simulink library "lib_accessory2"  (Simulink 10.1)
settings: Solver=VariableStepAuto  StartTime=0.0  StopTime=10.0  RelTol=1e-3
undefined symbols (not defined in the file or in its folder): acc_dcdc_eff, acc_elec_eff, acc_elec_efficiency, acc_elec_pwr, acc_mech_eff, acc_mech_pwr, acc_mech_trq, amb_tmp, ess_on, fc_on, map_spd, max_pwr, tc_gc_to_fc_ratio, time_step, vc_idle_bool, vc_idle_spd, vinf
undefined symbols (not defined in the file): acc_abc_dutycycle, acc_abc_init, acc_ac_dutycycle, acc_ac_init, acc_acdc_inverter_eff, acc_alt_init, acc_ef_dutycycle, acc_ef_init, acc_op_dutycycle, acc_op_init, acc_ps_dutycycle, acc_ps_init, acc_sindafile, acc_wp_dutycycle, acc_wp_init, generalName, logFlag
libraries: lib_cosimulation x29, $bdroot x15, lib_outputs x11, simulink3 x10, lib_accessory x8, lib_etc x2
(part 1 of 5)
settings Model: Creator=sateeshk  LastModifiedBy=sateeshk  ModifiedComment=abrooker -- Fri Jun 21 11:06:39 2002 -- Version 1.443
settings Model: ModifiedHistory=|
  | abrooker -- Fri Jun 21 11:06:39 2002 -- Version 1.443
  | 
  | 
  | abrooker -- Fri Jun 21 11:06:32 2002 -- Version 1.442
  | 
  | 
  | abrooker -- Fri Jun 21 11:03:06 2002 -- Version 1.441
  | 
  | 
  | abrooker -- Fri Jun 21 08:18:53 2002 -- Version 1.440
  | 
  | 
  | abrooker -- Fri Jun 21 08:07:14 2002 -- Version 1.439
  | 
  | 
  | abrooker -- Fri Jun 21 07:53:07 2002 -- Version 1.438
  | 
  | 
  | abrooker -- Thu Jun 20 15:33:10 2002 -- Version 1.437
  | 
  | 
  | abrooker -- Thu Jun 20 15:32:18 2002 -- Version 1.436
  | 
  | 
  | mokeefe -- Wed May 22 16:23:29 2002 -- Version 1.435
  | changed SindaTransAC model to take 5 outputs
  | 
  | mokeefe -- Thu Apr 18 08:24:09 2002 -- Version 1.434
  | saving the model:
  | o "without the model browser open"
  | o with only top-level screen visible
  | o with "fit to view" enabled
  | o with "status bar" off and "toolbar" off
  | o with "prompt to update model history with each save" on
  | 
  | tmarkel -- Mon Apr 15 11:38:46 2002 -- Version 1.428
  | 
  | 
  | tmarkel -- Mon Apr 15 11:38:46 2002 -- Version 1.428
  | 
  | 
  | tmarkel -- Mon Apr 15 11:38:36 2002 -- Version 1.427
  | 
  | 
  | mokeefe -- Mon Apr 15 11:36:55 2002 -- Version 1.426
  | added acc_sindafile variable into the SindaTransAC model
  | 
  | 
  | 
  | 
  | 
  | mokeefe -- Mon Apr 15 11:30:03 2002 -- Version 1.424
  | adding a feature to the sinda fluint s-function so that user can pass in the path to their executable file (*.im) function
  | 
  | 
  | abrooker -- Thu Apr 11 17:26:32 2002 -- Version 1.423
  | added vc_idle_bool in minimum fc shaft speed for stop/start:  otherwise
  | 
  | mokeefe -- Wed Apr 03 17:17:08 2002 -- Version 1.422
  | checked the configurable sub-system option for SindaTransAC
  | 
  | abrooker -- Tue Apr 02 08:21:35 2002 -- Version 1.421
  | 
  | 
  | abrooker -- Tue Apr 02 08:16:39 2002 -- Version 1.420
  | 
  | 
  | mokeefe -- Fri Mar 29 16:21:02 2002 -- Version 1.419
  | 
  | 
  | mokeefe -- Fri Mar 29 16:18:34 2002 -- Version 1.418
  | added SindaTransAC Sinda/Fluint cosim aux. model (transient air condition modeling)
  | 
  | mokeefe -- Fri Mar 29 09:01:44 2002 -- Version 1.417
  | 
  | 
  | mokeefe -- Fri Mar 29 09:00:29 2002 -- Version 1.416
  | 
  | 
  | mokeefe -- Fri Mar 29 08:55:21 2002 -- Version 1.415
  | 
  | 
  | mokeefe -- Fri Mar 29 08:54:32 2002 -- Version 1.414
  | 
  | 
  | mokeefe -- Fri Mar 29 08:34:07 2002 -- Version 1.413
  | 
  | 
  | mokeefe -- Fri Mar 29 08:33:22 2002 -- Version 1.412
  | rearranging the library for aesthetic purposes =)
  | 
  | mokeefe -- Fri Mar 29 08:27:44 2002 -- Version 1.411
  | took out two of the mechanical accessory options that will probably not be used (the same functionality is available with the remaining blocks). These blocks moved to the development subsystem for storage.
  | 
  | abrooker -- Thu Mar 28 16:18:46 2002 -- Version 1.410
  | (mokeefe) changed the Mechanical Accessory Load Driveline Block to use memory blocks for torque and power estimation (as opposed to two calculations)
  | 
  | abrooker -- Thu Mar 28 12:33:24 2002 -- Version 1.409
  | 
  | 
  | abrooker -- Thu Mar 28 12:25:41 2002 -- Version 1.408
  | 
  | 
  | abrooker -- Thu Mar 28 12:08:36 2002 -- Version 1.407
  | 
  | 
  | abrooker -- Thu Mar 28 12:04:18 2002 -- Version 1.406
  | 
  | 
  | abrooker -- Thu Mar 28 08:53:24 2002 -- Version 1.405
  | 
  | 
  | abrooker -- Thu Mar 28 08:49:44 2002 -- Version 1.404
  | 
  | 
  | mokeefe -- Wed Mar 27 07:38:24 2002 -- Version 1.403
  | 
  | 
  | mokeefe -- Wed Mar 27 07:37:49 2002 -- Version 1.402
  | added a masked variable (acc_max_spd) to the mechanical accessory loads library
  | 
  | mokeefe -- Wed Mar 20 10:22:56 2002 -- Version 1.401
  | changed the pictures for the configurable subsystem blocks to differentiate from the driveline blocks
  | 
  | mokeefe -- Tue Mar 12 13:44:43 2002 -- Version 1.400
  | 
  | 
  | mokeefe -- Tue Mar 12 13:36:01 2002 -- Version 1.399
  | cleaned up the library and reorganized block positions
  | 
  | 
  | mokeefe -- Tue Mar 12 13:34:33 2002 -- Version 1.398
  | 
  | 
  | mokeefe -- Tue Mar 12 13:34:15 2002 -- Version 1.397
  | 
  | 
  | mokeefe -- Tue Mar 12 13:29:31 2002 -- Version 1.396
  | 
  | 
  | mokeefe -- Tue Mar 12 13:25:46 2002 -- Version 1.395
  | 
  | 
  | mokeefe -- Tue Mar 12 13:09:55 2002 -- Version 1.394
  | changed the variable mechanical loads to include a water pump
  | 
  | mokeefe -- Tue Mar 12 12:07:07 2002 -- Version 1.393
  | 
  | 
  | mokeefe -- Tue Mar 12 12:06:03 2002 -- Version 1.392
  | 
  | 
  | mokeefe -- Tue Mar 12 12:04:31 2002 -- Version 1.391
  | 
  | 
  | mokeefe -- Tue Mar 12 11:59:22 2002 -- Version 1.390
  | 
  | 
  | mokeefe -- Tue Mar 12 11:54:25 2002 -- Version 1.389
  | changing the way that data signals are recorded (especially for the variable mechanical loads blocks--see SubLibraries/variable mechanical load --simulink implementation--)
  | 
  | mokeefe -- Fri Mar 08 07:13:02 2002 -- Version 1.388
  | added the tag acc_mech_pwr_est as a global tag to Mechanical Accessory Loads v2 <acc>
  | 
  | mokeefe -- Mon Mar 04 07:28:37 2002 -- Version 1.387
  | 
  | 
  | mokeefe -- Mon Mar 04 07:27:09 2002 -- Version 1.386
  | 
  | 
  | mokeefe -- Mon Mar 04 07:24:49 2002 -- Version 1.385
  | changed the mechanical accessory torque back to a simple version
  | 
  | mokeefe -- Fri Mar 01 16:40:21 2002 -- Version 1.384
  | 
  | 
  | mokeefe -- Fri Mar 01 16:37:19 2002 -- Version 1.383
  | 
  | 
  | mokeefe -- Fri Mar 01 15:08:33 2002 -- Version 1.382
  | 
  | 
  | mokeefe -- Fri Mar 01 12:12:06 2002 -- Version 1.381
  | 
  | 
  | mokeefe -- Fri Mar 01 12:10:27 2002 -- Version 1.380
  | 
  | 
  | mokeefe -- Fri Mar 01 11:39:14 2002 -- Version 1.379
  | 
  | 
  | mokeefe -- Fri Mar 01 11:20:41 2002 -- Version 1.378
  | 
  | 
  | mokeefe -- Fri Mar 01 10:50:57 2002 -- Version 1.377
  | 
  | 
  | mokeefe -- Fri Mar 01 10:18:24 2002 -- Version 1.376
  | 
  | 
  | mokeefe -- Fri Mar 01 10:16:01 2002 -- Version 1.375
  | 
  | 
  | mokeefe -- Fri Mar 01 10:13:39 2002 -- Version 1.374
  | 
  | 
  | mokeefe -- Fri Mar 01 09:58:45 2002 -- Version 1.373
  | 
  | 
  | mokeefe -- Fri Mar 01 09:31:13 2002 -- Version 1.372
  | 
  | 
  | mokeefe -- Fri Mar 01 09:30:34 2002 -- Version 1.371
  | 
  | 
  | mokeefe -- Fri Mar 01 09:00:19 2002 -- Version 1.370
  | 
  | 
  | mokeefe -- Fri Mar 01 08:27:00 2002 -- Version 1.369
  | 
  | 
  | mokeefe -- Fri Mar 01 08:04:14 2002 -- Version 1.368
  | 
  | 
  | mokeefe -- Thu Feb 28 08:51:52 2002 -- Version 1.367
  | 
  | 
  | mokeefe -- Thu Feb 28 08:48:14 2002 -- Version 1.366
  | 
  | 
  | mokeefe -- Thu Feb 28 08:21:55 2002 -- Version 1.365
  | 
  | 
  | mokeefe -- Thu Feb 28 08:20:46 2002 -- Version 1.364
  | adding an on/off flag for auxiliary systems to account for "engine off" states
  | 
  | mokeefe -- Thu Feb 28 08:10:24 2002 -- Version 1.363
  | 
  | 
  | mokeefe -- Wed Feb 27 14:38:39 2002 -- Version 1.362
  | 
  | 
  | mokeefe -- Wed Feb 27 14:34:06 2002 -- Version 1.361
  | 
  | 
  | mokeefe -- Wed Feb 27 14:33:33 2002 -- Version 1.360
  | 
  | 
  | mokeefe -- Wed Feb 27 14:29:19 2002 -- Version 1.359
  | 
  | 
  | mokeefe -- Wed Feb 27 14:12:33 2002 -- Version 1.358
  | 
  | 
  | mokeefe -- Wed Feb 27 14:11:56 2002 -- Version 1.357
  | 
  | 
  | mokeefe -- Wed Feb 27 14:06:17 2002 -- Version 1.356
  | 
  | 
  | mokeefe -- Wed Feb 27 14:04:01 2002 -- Version 1.355
  | added a "version 2" to mechanical auxiliary loads library which has a workaround that takes in the fc_spd_est instead of fc_spd_out_a--this enables vehicles to have an exact match between ADVISOR v3.2 and v2002
  | 
  | mokeefe -- Wed Feb 27 09:55:44 2002 -- Version 1.354
  | 
  | 
  | mokeefe -- Wed Feb 27 09:53:42 2002 -- Version 1.
  | 
  | mokeefe -- Tue Feb 26 15:16:41 2002 -- Version 1.352
  | 
  | 
  | mokeefe -- Tue Feb 26 14:01:11 2002 -- Version 1.351
  | 
  | 
  | mokeefe -- Tue Feb 26 13:25:47 2002 -- Version 1.350
  | 
  | 
  | mokeefe -- Tue Feb 26 10:40:53 2002 -- Version 1.349
  | 
  | 
  | mokeefe -- Mon Feb 25 16:05:53 2002 -- Version 1.348
  | 
  | 
  | mokeefe -- Mon Feb 25 15:35:04 2002 -- Version 1.347
  | 
  | 
  | mokeefe -- Mon Feb 25 15:33:00 2002 -- Version 1.346
  | 
  | 
  | mokeefe -- Mon Feb 25 15:26:23 2002 -- Version 1.345
  | 
  | 
  | mokeefe -- Mon Feb 25 15:24:36 2002 -- Version 1.344
  | 
  | 
  | mokeefe -- Mon Feb 25 15:23:19 2002 -- Version 1.343
  | 
  | 
  | mokeefe -- Mon Feb 25 15:19:58 2002 -- Version 1.342
  | 
  | 
  | mokeefe -- Mon Feb 25 15:17:22 2002 -- Version 1.341
  | 
  | 
  | mokeefe -- Mon Feb 25 15:04:08 2002 -- Version 1.340
  | 
  | 
  | mokeefe -- Mon Feb 25 14:59:43 2002 -- Version 1.339
  | 
  | 
  | mokeefe -- Mon Feb 25 14:50:11 2002 -- Version 1.338
  | 
  | 
  | mokeefe -- Mon Feb 25 14:37:23 2002 -- Version 1.337
  | 
  | 
  | mokeefe -- Mon Feb 25 14:24:02 2002 -- Version 1.336
  | 
  | 
  | mokeefe -- Mon Feb 25 14:19:40 2002 -- Version 1.335
  | 
  | 
  | mokeefe -- Mon Feb 25 14:14:18 2002 -- Version 1.334
  | 
  | 
  | mokeefe -- Mon Feb 25 14:09:13 2002 -- Version 1.333
  | 
  | 
  | mokeefe -- Mon Feb 25 13:38:54 2002 -- Version 1.332
  | 
  | 
  | mokeefe -- Mon Feb 25 13:38:02 2002 -- Version 1.331
  | 
  | 
  | mokeefe -- Wed Feb 20 09:52:02 2002 -- Version 1.330
  | 
  | 
  | mokeefe -- Wed Feb 20 09:49:29 2002 -- Version 1.329
  | changed the acc_mech_trq_a, acc_mech_pwr_a, acc_mech_trq_r, acc_mech_pwr_r, acc_elec_pwr_a, acc_elec_pwr_r GOTO blocks to global scope.
  | 
  | mokeefe -- Wed Feb 20 09:47:28 2002 -- Version 1.328
  | 
  | 
  | mokeefe -- Wed Feb 20 09:46:46 2002 -- Version 1.327
  | 
  | 
  | mokeefe -- Wed Feb 20 07:42:37 2002 -- Version 1.326
  | 
  | 
  | mokeefe -- Wed Feb 20 07:42:12 2002 -- Version 1.325
  | 
  | 
  | mokeefe -- Wed Feb 20 07:41:46 2002 -- Version 1.324
  | 
  | 
  | mokeefe -- Tue Feb 19 16:34:31 2002 -- Version 1.323
  | 
  | 
  | mokeefe -- Tue Feb 19 16:31:37 2002 -- Version 1.322
  | 
  | 
  | mokeefe -- Tue Feb 19 16:28:38 2002 -- Version 1.321
  | changed the accessory GOTO tags to global scope in Electrical Accessory Loads
  | 
  | mokeefe -- Tue Feb 19 16:14:33 2002 -- Version 1.320
  | first release to RCS
  | 
  | mokeefe -- Tue Feb 19 16:12:28 2002 -- Version 1.319
  | 
  | 
  | mokeefe -- Tue Feb 19 16:06:11 2002 -- Version 1.318
  | 
  | 
  | mokeefe -- Tue Feb 19 16:02:32 2002 -- Version 1.317
  | 
  | 
  | mokeefe -- Tue Feb 19 15:58:43 2002 -- Version 1.316
  | 
  | 
  | mokeefe -- Tue Feb 19 15:55:41 2002 -- Version 1.315
  | 
  | 
  | mokeefe -- Tue Feb 19 15:53:46 2002 -- Version 1.314
  | 
  | 
  | mokeefe -- Tue Feb 19 15:49:12 2002 -- Version 1.313
  | 
  | 
  | mokeefe -- Tue Feb 19 15:42:48 2002 -- Version 1.312
  | 
  | 
  | mokeefe -- Tue Feb 19 15:41:05 2002 -- Version 1.311
  | 
  | 
  | mokeefe -- Tue Feb 19 15:38:40 2002 -- Version 1.310
  | 
  | 
  | mokeefe -- Tue Feb 19 15:28:06 2002 -- Version 1.309
  | 
  | 
  | mokeefe -- Tue Feb 19 15:18:02 2002 -- Version 1.308
  | 
  | 
  | mokeefe -- Tue Feb 19 14:53:21 2002 -- Version 1.307
  | 
  | 
  | mokeefe -- Tue Feb 19 14:46:24 2002 -- Version 1.306
  | 
  | 
  | mokeefe -- Tue Feb 19 14:20:08 2002 -- Version 1.305
  | 
  | 
  | mokeefe -- Tue Feb 19 14:15:36 2002 -- Version 1.304
  | 
  | 
  | mokeefe -- Tue Feb 19 13:24:42 2002 -- Version 1.303
  | 
  | 
  | mokeefe -- Tue Feb 19 13:17:05 2002 -- Version 1.302
  | 
  | 
  | mokeefe -- Tue Feb 19 13:11:20 2002 -- Version 1.301
  | 
  | 
  | mokeefe -- Tue Feb 19 11:29:38 2002 -- Version 1.300
  | 
  | 
  | mokeefe -- Tue Feb 19 11:24:45 2002 -- Version 1.299
  | adding electrical accessory block
  | 
  | 
  | mokeefe -- Tue Feb 19 10:53:36 2002 -- Version 1.298
  | 
  | 
  | mokeefe -- Tue Feb 19 10:19:54 2002 -- Version 1.297
  | added electrical accessory loads block
  | 
  | 
  | mokeefe -- Thu Feb 14 17:56:03 2002 -- Version 1.296
  | 
  | 
  | mokeefe -- Thu Feb 14 17:54:33 2002 -- Version 1.295
  | 
  | 
  | mokeefe -- Thu Feb 14 17:51:07 2002 -- Version 1.294
  | 
  | 
  | mokeefe -- Thu Feb 14 17:49:19 2002 -- Version 1.293
  | changing the way that data is "logged" to displays and scopes vs. workspace on some components that I expect will have to be used multiple times... (a workaround for now)
  | 
  | mokeefe -- Thu Feb 14 17:21:35 2002 -- Version 1.292
  | 
  | 
  | mokeefe -- Thu Feb 14 16:55:33 2002 -- Version 1.291
  | 
  | 
  | mokeefe -- Thu Feb 14 16:21:30 2002 -- Version 1.290
  | 
  | 
  | mokeefe -- Thu Feb 14 16:19:08 2002 -- Version 1.289
  | 
  | 
  | mokeefe -- Thu Feb 14 16:17:00 2002 -- Version 1.288
  | 
  | 
  | mokeefe -- Thu Feb 14 16:15:50 2002 -- Version 1.287
  | 
  | 
  | mokeefe -- Thu Feb 14 16:14:24 2002 -- Version 1.286
  | 
  | 
  | mokeefe -- Thu Feb 14 16:13:43 2002 -- Version 1.285
  | 
  | 
  | mokeefe -- Thu Feb 14 15:43:46 2002 -- Version 1.284
  | 
  | 
  | mokeefe -- Thu Feb 14 15:42:22 2002 -- Version 1.283
  | 
  | 
  | mokeefe -- Thu Feb 14 15:31:24 2002 -- Version 1.282
  | 
  | 
  | mokeefe -- Thu Feb 14 15:26:13 2002 -- Version 1.281
  | 
  | 
  | mokeefe -- Thu Feb 14 15:25:37 2002 -- Version 1.280
  | 
  | 
  | mokeefe -- Thu Feb 14 15:19:19 2002 -- Version 1.279
  | 
  | 
  | mokeefe -- Thu Feb 14 15:10:41 2002 -- Version 1.278
  | 
  | 
  | mokeefe -- Thu Feb 14 14:28:51 2002 -- Version 1.277
  | 
  | 
  | mokeefe -- Thu Feb 14 14:26:34 2002 -- Version 1.276
  | 
  | 
  | mokeefe -- Thu Feb 14 10:50:49 2002 -- Version 1.275
  | 
  | 
  | mokeefe -- Thu Feb 14 10:47:05 2002 -- Version 1.274
  | 
  | 
  | mokeefe -- Thu Feb 14 10:40:54 2002 -- Version 1.273
  | 
  | 
  | mokeefe -- Thu Feb 14 10:23:01 2002 -- Version 1.272
  | 
  | 
  | mokeefe -- Thu Feb 14 10:05:05 2002 -- Version 1.271
  | 
  | 
  | mokeefe -- Thu Feb 14 09:56:25 2002 -- Version 1.270
  | 
  | 
  | mokeefe -- Thu Feb 14 09:55:54 2002 -- Version 1.269
  | changed the "signal width" parameters of blocks such that they work correctly
  | 
  | mokeefe -- Thu Feb 14 09:54:47 2002 -- Version 1.268
  | 
  | 
  | mokeefe -- Thu Feb 14 09:51:13 2002 -- Version 1.267
  | 
  | 
  | mokeefe -- Thu Feb 14 08:58:02 2002 -- Version 1.266
  | 
  | 
  | mokeefe -- Thu Feb 14 08:39:00 2002 -- Version 1.265
  | changed the port width in alternator block back to dynamically sized
  | 
  | 
  | mokeefe -- Thu Feb 14 08:06:18 2002 -- Version 1.264
  | 
  | 
  | mokeefe -- Wed Feb 13 16:52:46 2002 -- Version 1.263
  | adding signal specification blocks to force the size of signals
  | 
  | mokeefe -- Wed Feb 13 16:52:26 2002 -- Version 1.262
  | 
  | 
  | mokeefe -- Wed Feb 13 16:46:44 2002 -- Version 1.261
  | 
  | 
  | mokeefe -- Wed Feb 13 16:31:21 2002 -- Version 1.260
  | 
  | 
  | mokeefe -- Wed Feb 13 16:30:50 2002 -- Version 1.259
  | 
  | 
  | mokeefe -- Wed Feb 13 16:25:26 2002 -- Version 1.258
  | 
  | 
  | mokeefe -- Wed Feb 13 15:56:34 2002 -- Version 1.257
  | testing
  | 
  | 
  | mokeefe -- Wed Feb 13 14:44:42 2002 -- Version 1.256
  | the accessory library

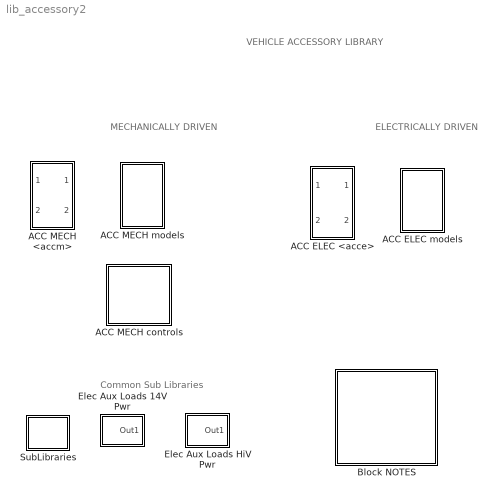
== system lib_accessory2 ==
  note: Common Sub Libraries
  note: VEHICLE ACCESSORY LIBRARY
  note: MECHANICALLY DRIVEN
  note: ELECTRICALLY DRIVEN
  ACC ELEC models : Subsystem
  ACC ELEC <acce> : Subsystem  mask(Stand-Alone Electrical Accessory Mask){generalName='acc', logPick=Log, initFileName={}, modCell={}, imgFileName='bdi_acc_elec.bmp', DEBUG=OFF}
      mask prompts: generalName "General Name of this Component [char]"; logPick "Log Variables to Workspace?"; initFileName "Initialization File(s) [cell array of char]"; modCell "Modification Cell [2 column cell array of param and val]"; imgFileName "Icon image file name [char--evaluated]"
      mask init:
      | % initialization via m-file script
      | advSACompMaskInit;
      mask TypeOptions logPick: Don't Log | Log
      mask TypeOptions DEBUG: ON | OFF
      mask Display: image(imread(imgFileName))
  ACC MECH controls : Subsystem
  ACC MECH models : Subsystem
  ACC MECH <accm> : Subsystem  mask(Stand-Alone Mechanical Accessory Mask){generalName='acc', logPick=Log, initFileName={}, modCell={}, imgFileName='bdi_acc_pic.bmp', DEBUG=OFF}
      mask prompts: generalName "General Name of this Component [char]"; logPick "Log Variables to Workspace?"; initFileName "Initialization File(s) [cell array of char]"; modCell "Modification Cell [2 column cell array of param and val]"; imgFileName "Icon image file name [char--evaluated]"
      mask init:
      | % initialization via m-file script
      | advSACompMaskInit;
      mask TypeOptions logPick: Don't Log | Log
      mask TypeOptions DEBUG: ON | OFF
      mask Display: image(imread(imgFileName))
  Block NOTES : Subsystem
      mask Display: disp('Model\nNOTES')
  Elec Aux Loads 14V Pwr : Subsystem
  Elec Aux Loads HiV Pwr : Subsystem
  SubLibraries : Subsystem

== system lib_accessory2/ACC ELEC models ==
  note: Electrical Auxiliary System Models
  note: configurable subsystem template
  note: Electrical Power
      | Consumption (W)
  Electrical Accessories: Constant : Subsystem
      mask Display: image(imread('bdi_acc_elec_cs.bmp'))
  Electrical Accessories: Time Variable : Subsystem
      mask Display: image(imread('bdi_acc_elec_cs.bmp'))
  electrical accessories (W) : Subsystem  BlockChoice=Electrical Accessories: Time Variable
      settings: TemplateBlock=self  MemberBlocks=Electrical Accessories: Constant,Electrical Accessories: Time Variable
      mask Display: image(imread('bdi_acc_elec_cs.bmp'))

== system lib_accessory2/ACC ELEC <acce> ==
  note: ELECTRICAL ACCESSORY
      | Interface
  elec pwr out r (W) : Inport
  elec pwr in a (W) : Inport  Port=2
  ACC ELEC model and interface : Subsystem
      mask Display: image(imread('bdi_acc_elec.bmp'))
  elec pwr in r (W) : Outport
  elec pwr out a (W) : Outport  Port=2
  tag scope: accReqOut=global, accSensors=global
  wires:
  [accControl] -> ACC ELEC model and interface/3(control)
  elec pwr out r (W)/1 -> ACC ELEC model and interface/1("requested electrical Power, out to the driveline (W)")
  elec pwr in a (W)/1 -> ACC ELEC model and interface/2(achieved power in from power source (W))
  ACC ELEC model and interface/1(requested out) -> [accReqOut]
  ACC ELEC model and interface/2("requested electrical Power, in from the power source (W)") -> elec pwr in r (W)/1
  ACC ELEC model and interface/3("achieved electrical Power, out to the driveline (W)") -> elec pwr out a (W)/1
  ACC ELEC model and interface/4(sensors) -> [accSensors]

== system lib_accessory2/ACC MECH controls ==
  Mechanical Accessories : Subsystem

== system lib_accessory2/ACC MECH models ==
  note: Mechanical Auxiliary System Models
  note: These configurable sub-systems
      | are associated with the above model
  Mechanical Accessories: Const Mech Var Elect : Subsystem
      mask Display: image(imread('bdi_acc_pic_cs.bmp'))
  Mechanical Accessories: Constant Mechanical & Electrical : Subsystem
      mask Display: image(imread('bdi_acc_pic_cs.bmp'))
  Mechanical Accessories: Speed Dependant and Variable Electrical : Subsystem
      mask Display: image(imread('bdi_acc_pic_cs.bmp'))
  Saber Dual Voltage Cosim : Subsystem
      mask Display: image(imread('bdi_acc_pic_cs.bmp'))
  Saber Single Voltage Cosim : Subsystem
      mask Display: image(imread('bdi_acc_pic_cs.bmp'))
  SindaTransAC : Subsystem
      mask Display: image(imread('bdi_acc_pic_cs.bmp'))
  mechanical accessories (Nm) : Subsystem  BlockChoice=Mechanical Accessories: Const Mech Var Elect
      settings: TemplateBlock=self  MemberBlocks=Mechanical Accessories: Const Mech Var Elect,Mechanical Accessories: Constant Mechanical & Electrical,Mechanical Accessories: Speed Dependant and Variable Electrical,Saber Dual Voltage Cosim,Saber Single Voltage Cosim,SindaTransAC
      mask Display: image(imread('bdi_acc_pic_cs.bmp'))

== system lib_accessory2/ACC MECH <accm> ==
  note: MECHANICAL ACCESSORY
      | Interface
  trq and spd out requested : Inport
  trq and spd in achieved : Inport  Port=2
  mechanical accessory model and interface : Subsystem  AncestorBlock=lib_accessory2/ACC MECH <accm>/mechanical accessory model and interface
  trq and spd in  requested : Outport
  "trq and spd out achieved " : Outport  Port=2
  tag scope: accReqOut=global, accSensors=global
  wires:
  mechanical accessory model and interface/3("T, w out achieved") -> "trq and spd out achieved "/1
  trq and spd in achieved/1 -> mechanical accessory model and interface/2("T, w in achieved")
  trq and spd out requested/1 -> mechanical accessory model and interface/1("T, w out requested")
  mechanical accessory model and interface/2(T,w in request) -> trq and spd in  requested/1
  mechanical accessory model and interface/1(Out Request) -> [accReqOut]
  [accControl] -> mechanical accessory model and interface/3(control)
  mechanical accessory model and interface/4(sensors) -> [accSensors]

== system lib_accessory2/Block NOTES ==
  note: The accessory library defines ADVISOR driveline blocks and their submodels/subsystems having
      | to do with mechanical and electrical auxiliary loads. Note that time-variable electrical load
      | models are defined in sublib_models.mdl (a library file)
  note: Each driveline block takes in a power or torque/speed request and augments that request
      | up the driveline toward the prime mover or power generator. On the way down, the power use
      | is re-accounted such that only the driveline energy is sent. The basic assumption is that auxiliary
      | loads are satisfied first and then power is sent down the driveline. Users may wish to implement their
      | own custom control strategies if this is not the case.
  note: This library uses configurable subsystems extensively to maximize the basic interfaces and
      | isolate the things that change from the things that stay the same. Configurable subsystems
      | are added to the model by clicking on the configurable subsystem block template (outlined in blue)
      | and checking the box next to the model name you would like to add.
  note: load_on is used as a flag in the models to switch aux loads on and off
  note: "Mechanical Loads" and "Electrical Loads" are distinguised by what form of energy
      | would have to pass the boundary of the auxiliary system model to power the
      | accessory loads. For example, a mechanical load may have electrical loads and
      | an alternator built into the model. However, if shaft energy must be supplied to
      | power the mechanical load, then the load is considered a Mechanical load because
      | it requires the shaft power as an input to the auxiliary model.
      |
      | Conversely, a load that feeds off of a power bus would be termed an electrical load

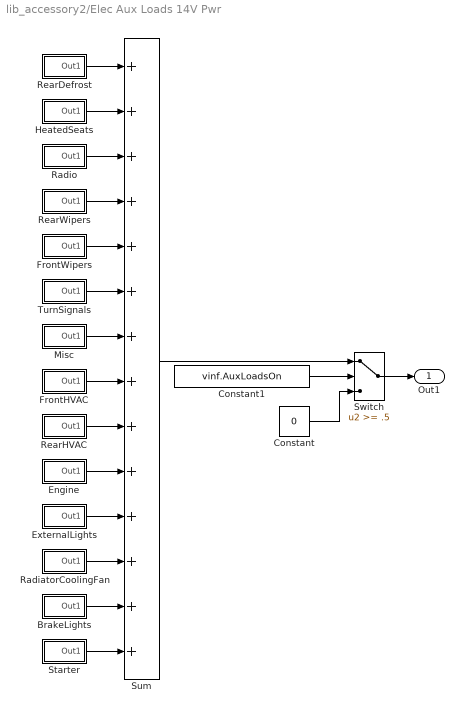
== system lib_accessory2/Elec Aux Loads 14V Pwr ==
  BrakeLights : Subsystem
  Constant : Constant  Value=0
  Constant1 : Constant  Value=vinf.AuxLoadsOn
  Engine : Subsystem
  ExternalLights : Subsystem
  FrontHVAC : Subsystem
  FrontWipers : Subsystem
  HeatedSeats : Subsystem
  Misc : Subsystem
  RadiatorCoolingFan : Subsystem
  Radio : Subsystem
  RearDefrost : Subsystem
  RearHVAC : Subsystem
  RearWipers : Subsystem
  Starter : Subsystem
  Sum : Sum  Inputs=++++++++++++++  SaturateOnIntegerOverflow=on
  Switch : Switch  Threshold=.5  SaturateOnIntegerOverflow=on  InputSameDT=on
  TurnSignals : Subsystem
  Out1 : Outport
  wires:
  Starter/1(Out1) -> Sum/14
  BrakeLights/1(Out1) -> Sum/13
  RadiatorCoolingFan/1(Out1) -> Sum/12
  ExternalLights/1(Out1) -> Sum/11
  Engine/1(Out1) -> Sum/10
  RearHVAC/1(Out1) -> Sum/9
  FrontHVAC/1(Out1) -> Sum/8
  Misc/1(Out1) -> Sum/7
  TurnSignals/1(Out1) -> Sum/6
  FrontWipers/1(Out1) -> Sum/5
  RearWipers/1(Out1) -> Sum/4
  Radio/1(Out1) -> Sum/3
  HeatedSeats/1(Out1) -> Sum/2
  RearDefrost/1(Out1) -> Sum/1
  Constant1/1 -> Switch/2
  Constant/1 -> Switch/3
  Sum/1 -> Switch/1
  Switch/1 -> Out1/1

== system lib_accessory2/Elec Aux Loads HiV Pwr ==
  Constant : Constant  Value=0
  Constant1 : Constant  Value=vinf.AuxLoadsOn
  CurrentLoad1 : Subsystem
  PowerLoad1 : Subsystem
  PowerLoad2 : Subsystem
  PowerLoad3 : Subsystem
  SpeedLoad1 : Subsystem
  Starter : Subsystem
  Sum : Sum  Inputs=++++++  SaturateOnIntegerOverflow=on
  Switch : Switch  Threshold=.5  SaturateOnIntegerOverflow=on  InputSameDT=on
  Out1 : Outport
  wires:
  Switch/1 -> Out1/1
  Constant/1 -> Switch/3
  Constant1/1 -> Switch/2
  PowerLoad1/1(Out1) -> Sum/1
  PowerLoad2/1(Out1) -> Sum/2
  PowerLoad3/1(Out1) -> Sum/3
  CurrentLoad1/1(Out1) -> Sum/4
  SpeedLoad1/1(Out1) -> Sum/5
  Starter/1(Out1) -> Sum/6
  Sum/1 -> Switch/1

== system lib_accessory2/SubLibraries ==
  note: Conventional Mechanical
      | Auxiliary Load System
  note: duty cycle (1=full on, 0=off)
  note: required power (W)
  note: Auxiliary Device:
      | Power as a function of
      | * Instantaneous Shaft Speed (rad/s) and
      | * Time Dependant (Normalized) Load (i.e., duty cycle)
  note: shaft speed (rad/s)
  note: time (s)
  note: Auxiliary Device
      | Models
  note: Auxiliary Device:
      | Power as a function of
      | * Instantaneous Shaft Speed (rad/s) and
      | * Instantaneous Load (W)
  note: ----------------------------------------------------------------------------------
  note: shaft speed (rad/s)
  note: load on device (W)
  note: required power (W)
  note: m-file lookup
  note: ----------------------------------------------------------------------------------
  note: Auxiliary Device:
      | Power as a function of
      | * Instantaneous Shaft Speed (rad/s) and
      | * Time Dependant (Normalized) Load (i.e., duty cycle)
  note: Simulink Implementation
  note: shaft speed (rad/s)
  note: time (s)
  note: duty cycle (1=full on, 0=off)
  note: required power (W)
  note: ----------------------------------------------------------------------------------
  note: Simulink Implementation
  note: Auxiliary Device:
      | Power as a function of
      | * Instantaneous Shaft Speed (rad/s) and
      | * Time Dependant (Normalized) Load (i.e., duty cycle)
  note: Data Loggers
  Shaft Speed and Actual Load Auxiliary Device : Subsystem  mask{conv_eff=, pwr_func=}
      mask prompts: conv_eff "Load Constant Conversion Efficiency (decimal 0<=eff<=1)"; pwr_func "Variable holding string of Power Function Name"
  Shaft Speed and Actual Load Auxiliary Device--lookuptable : Subsystem  mask{conv_eff=, fname=}
      mask prompts: conv_eff "Load Constant Conversion Efficiency (decimal 0<=eff<=1)"; fname "Initialization M-File"
      mask init:
      | eval(fname);
      | maxSpd=max(map_spd);
      | minSpd=min(map_spd);
  Shaft Speed and Time Loaded Auxiliary Device : Subsystem  mask{acc_duty=, pwr_func=}
      mask prompts: acc_duty "Accessory duty cycle vs. time (2 Col: [time, duty])"; pwr_func "Variable holding string of Power Function Name"
  Shaft Speed and Time Loaded Auxiliary Device--lookuptable : Subsystem  mask{fname=, acc_duty=}
      mask prompts: fname "Initialization M-File"; acc_duty "Accessory Duty Cycle (1st Col is time, 2nd Column is load fraction)"
      mask init:
      | eval(fname); % load the script function
      | maxSpd=max(map_spd);
      | minSpd=min(map_spd);
      mask Help:
      | <p>This block must contain a variable of the string of an m-file for initialization:</p>
      | 
      | <ul>
      | <li>e.g., 'myMfile' or fileName (where fileName='myMfile')</li>
      | </ul>
      | 
      | <p>The initialization m-file must contain the variables:
      | <ol>
      | <li>map_spd</li>, <li>map_load</li>, and <li>pwr_map</li>
      | </ol>
      | 
      | <p>In addition, the user must specify a matrix with the auxiliary duty cycle. This matrix is a two column matrix with time values in the first column and load fraction in the second column. Load fraction is a value from 0 to 1 which tells weather a device is "full off" "full on" or somewhere in between.</p>
      | 
      | <p>created 7 February 2002 by mpo at NREL</p>
  accessory mechanical torque and power calcs (Nm) : Subsystem
  data logging probes dummy : Subsystem
  data logging probes for conventional mechanical loads : Subsystem
  data probes : Subsystem  BlockChoice=data logging probes for conventional mechanical loads
      settings: TemplateBlock=self  MemberBlocks=data logging probes dummy,data logging probes for conventional mechanical loads
  electrical power logging : Subsystem  mask{eff=acc_mech_eff}
      mask prompts: eff "efficiency of accessory systems (decimal)"
  mechanical power logging : Subsystem  mask{eff=acc_mech_eff}
      mask prompts: eff "efficiency of accessory systems (decimal)"
  variable mechanical load --simulink implementation-- : Subsystem
  variable mechanical load --simulink implementation-- no alternator : Subsystem

== system lib_accessory2/ACC ELEC models/Electrical Accessories: Constant ==
  note: (W)
  Constant : Constant  Value=acc_elec_pwr/acc_elec_efficiency
  P_elec_acc : Outport  InitialOutput=0
  wires:
  Constant/1 -> P_elec_acc/1

== system lib_accessory2/ACC ELEC models/Electrical Accessories: Time Variable ==
  note: (W)
  Constant : Constant  Value=acc_elec_pwr
  Elec Aux Loads 14V Pwr : $bdroot/Elec Aux Loads 14V Pwr
      settings: RTWFcnNameOpts=Auto  RTWFileNameOpts=Auto
  Elec Aux Loads HiV Pwr : $bdroot/Elec Aux Loads HiV Pwr
      settings: RTWFcnNameOpts=Auto  RTWFileNameOpts=Auto
  Sum : Sum  Inputs=+++  SaturateOnIntegerOverflow=on
  dcdc converter : Gain  Gain=1/acc_dcdc_eff  SaturateOnIntegerOverflow=on
  divide by eff : Gain  Gain=1/acc_elec_eff  SaturateOnIntegerOverflow=on
  P_elec_acc : Outport  InitialOutput=0
  wires:
  Elec Aux Loads 14V Pwr/1 -> dcdc converter/1
  Sum/1 -> divide by eff/1
  divide by eff/1 -> P_elec_acc/1
  Constant/1 -> Sum/1
  dcdc converter/1 -> Sum/2
  Elec Aux Loads HiV Pwr/1 -> Sum/3

== system lib_accessory2/ACC ELEC models/electrical accessories (W) ==
  Electrical Accessories: Time Variable : lib_accessory/Electrical Accessories: Time Variable
  P_elec_acc : Outport
  wires:
  Electrical Accessories: Time Variable/1 -> P_elec_acc/1

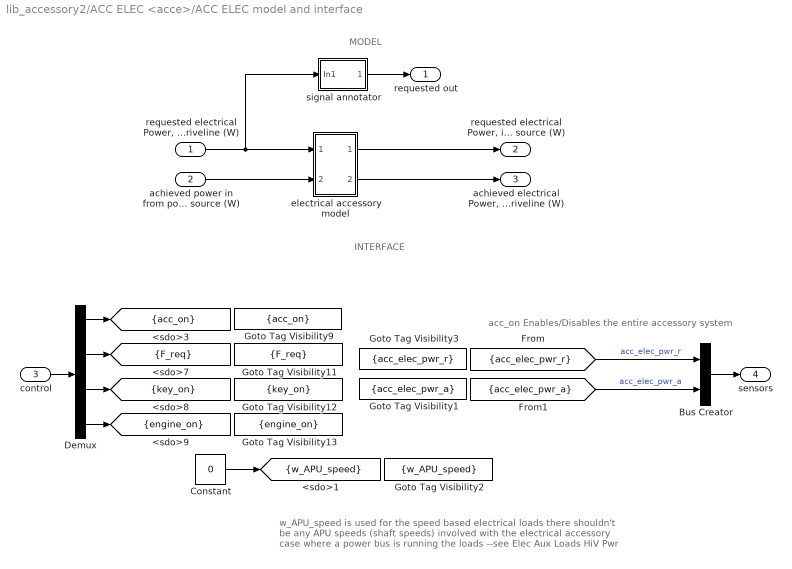
== system lib_accessory2/ACC ELEC <acce>/ACC ELEC model and interface ==
  note: INTERFACE
  note: acc_on Enables/Disables the entire accessory system
  note: MODEL
  note: w_APU_speed is used for the speed based electrical loads
      | there shouldn't be any APU speeds (shaft speeds) involved with
      | the electrical accessory case where a power bus is running the loads
      | --see Elec Aux Loads HiV Pwr
  "requested electrical Power, out to the driveline (W)" : Inport
  achieved power in from power source (W) : Inport  Port=2
  control : Inport  Port=3
  Bus Creator : BusCreator  Inputs=2
  Constant : Constant  Value=0
  Demux : Demux
  Goto Tag Visibility1 : GotoTagVisibility  GotoTag=acc_elec_pwr_a
  Goto Tag Visibility11 : GotoTagVisibility  GotoTag=F_req
  Goto Tag Visibility12 : GotoTagVisibility  GotoTag=key_on
  Goto Tag Visibility13 : GotoTagVisibility  GotoTag=engine_on
  Goto Tag Visibility2 : GotoTagVisibility  GotoTag=w_APU_speed
  Goto Tag Visibility3 : GotoTagVisibility  GotoTag=acc_elec_pwr_r
  Goto Tag Visibility9 : GotoTagVisibility  GotoTag=acc_on
  electrical accessory model : Subsystem
  signal annotator : Subsystem
  requested out : Outport
  "requested electrical Power, in from the power source (W)" : Outport  Port=2
  "achieved electrical Power, out to the driveline (W)" : Outport  Port=3
  sensors : Outport  Port=4
  tag scope: F_req=scoped, acc_on=scoped, engine_on=scoped, key_on=scoped, w_APU_speed=scoped
  wires:
  "requested electrical Power, out to the driveline (W)"/1 -> electrical accessory model/1("requested electrical Power, out to the driveline (W)"), signal annotator/1(In1)
  electrical accessory model/1("requested electrical Power, in from the power source (W)") -> "requested electrical Power, in from the power source (W)"/1
  achieved power in from power source (W)/1 -> electrical accessory model/2(achieved power in from power source (W))
  electrical accessory model/2("achieved electrical Power, out to the driveline (W)") -> "achieved electrical Power, out to the driveline (W)"/1
  Demux/1 -> [acc_on]
  Demux/2 -> [F_req]
  [acc_elec_pwr_r] -> Bus Creator/1  "acc_elec_pwr_r"
  [acc_elec_pwr_a] -> Bus Creator/2  "acc_elec_pwr_a"
  Demux/3 -> [key_on]
  Demux/4 -> [engine_on]
  Bus Creator/1 -> sensors/1
  control/1 -> Demux/1
  signal annotator/1(Out1) -> requested out/1
  Constant/1 -> [w_APU_speed]

== system lib_accessory2/ACC MECH controls/Mechanical Accessories ==
  Bus Creator : BusCreator  Inputs=9
  Bus Selector : BusSelector  OutputSignals=fc_spd_est
  Bus Selector1 : BusSelector  OutputSignals=F_req
  Bus Selector2 : BusSelector  OutputSignals=key_on
  Bus Selector3 : BusSelector  OutputSignals=engine_on
  Constant : Constant  Value=not(ess_on)*1
  Constant1 : Constant  Value=inf
  Constant2 : Constant  Value=(vc_idle_spd*vc_idle_bool)+eps
  mechanical accessory controller : Subsystem
  tag scope: accControl=global
  wires:
  Constant1/1 -> mechanical accessory controller/2(maximum accessory speed)
  Constant2/1 -> mechanical accessory controller/3(minimum accessory speed)
  Constant/1 -> mechanical accessory controller/4(electrical accessories on?)
  mechanical accessory controller/1(acc_on) -> Bus Creator/1
  mechanical accessory controller/2(acc_mech_spd_r) -> Bus Creator/2
  mechanical accessory controller/3(acc_mech_spd_a) -> Bus Creator/3
  mechanical accessory controller/4(acc_max_spd) -> Bus Creator/4
  mechanical accessory controller/5(acc_min_spd) -> Bus Creator/5
  mechanical accessory controller/6(elec_acc_on_bool) -> Bus Creator/6
  mechanical accessory controller/7(F_req) -> Bus Creator/7
  mechanical accessory controller/8(key_on) -> Bus Creator/8
  mechanical accessory controller/9(engine_on) -> Bus Creator/9
  Bus Creator/1 -> [accControl]
  [fcControl] -> Bus Selector2/1
  Bus Selector2/1 -> mechanical accessory controller/6(key on?)  "<key_on>"
  [fcControl] -> Bus Selector3/1
  Bus Selector3/1 -> mechanical accessory controller/7(engine on?)  "<engine_on>"
  [fcReqOut] -> Bus Selector/1
  Bus Selector/1 -> mechanical accessory controller/1(accessory reference shaft speed)  "<fc_spd_est>"
  [vehReqOut] -> Bus Selector1/1
  Bus Selector1/1 -> mechanical accessory controller/5(Force required for vehicle motion)  "<F_req>"

== system lib_accessory2/ACC MECH models/Mechanical Accessories: Const Mech Var Elect ==
  note: engine shaft speed
  note: (Nm)
  note: (W)
  w_APU : Inport
  Constant : Constant  Value=acc_mech_pwr
  Constant1 : Constant  Value=acc_mech_trq
  Constant2 : Constant  Value=acc_elec_pwr
  Elec Aux Loads 14V Pwr : $bdroot/Elec Aux Loads 14V Pwr
      settings: RTWFcnNameOpts=Auto  RTWFileNameOpts=Auto
  Elec Aux Loads HiV Pwr : $bdroot/Elec Aux Loads HiV Pwr
      settings: RTWFcnNameOpts=Auto  RTWFileNameOpts=Auto
  Mux : Mux  Inputs=3
  Product : Product  SaturateOnIntegerOverflow=on
  Sum1 : Sum  Inputs=+++  SaturateOnIntegerOverflow=on
  accessory mechanical torque and power calcs (Nm) : $bdroot/SubLibraries/accessory mechanical torque and power calcs (Nm)
      settings: RTWFcnNameOpts=Auto  RTWFileNameOpts=Auto
  dcdc converter : Gain  Gain=1/acc_dcdc_eff  SaturateOnIntegerOverflow=on
  T_acc : Outport  InitialOutput=0
  P_mech_acc : Outport  Port=2  InitialOutput=0
  wires:
  w_APU/1 -> accessory mechanical torque and power calcs (Nm)/1
  accessory mechanical torque and power calcs (Nm)/1 -> T_acc/1
  accessory mechanical torque and power calcs (Nm)/2 -> P_mech_acc/1
  Mux/1 -> accessory mechanical torque and power calcs (Nm)/2
  Constant/1 -> Mux/1
  Constant1/1 -> Mux/2
  Product/1 -> Mux/3
  [elec_acc_on_bool] -> Product/2
  Elec Aux Loads 14V Pwr/1 -> dcdc converter/1
  Constant2/1 -> Sum1/1
  Sum1/1 -> Product/1
  dcdc converter/1 -> Sum1/2
  Elec Aux Loads HiV Pwr/1 -> Sum1/3

== system lib_accessory2/ACC MECH models/Mechanical Accessories: Constant Mechanical & Electrical ==
  note: engine shaft speed
  note: (Nm)
  note: (W)
  w_APU : Inport
  Constant : Constant  Value=acc_mech_pwr
  Constant1 : Constant  Value=acc_mech_trq
  Constant2 : Constant  Value=acc_elec_pwr
  Mux : Mux  Inputs=3
  Product : Product  SaturateOnIntegerOverflow=on
  accessory mechanical torque and power calcs (Nm) : $bdroot/SubLibraries/accessory mechanical torque and power calcs (Nm)
      settings: RTWFcnNameOpts=Auto  RTWFileNameOpts=Auto
  T_acc : Outport  InitialOutput=0
  P_mech_acc : Outport  Port=2  InitialOutput=0
  wires:
  w_APU/1 -> accessory mechanical torque and power calcs (Nm)/1
  accessory mechanical torque and power calcs (Nm)/1 -> T_acc/1
  accessory mechanical torque and power calcs (Nm)/2 -> P_mech_acc/1
  Mux/1 -> accessory mechanical torque and power calcs (Nm)/2
  Constant/1 -> Mux/1
  Constant1/1 -> Mux/2
  Constant2/1 -> Product/1
  Product/1 -> Mux/3
  [elec_acc_on_bool] -> Product/2

== system lib_accessory2/ACC MECH models/Mechanical Accessories: Speed Dependant and Variable Electrical ==
  note: engine shaft speed
  note: (Nm)
  note: (W)
  w_APU : Inport
  Constant1 : Constant  Value=acc_elec_pwr
  Constant2 : Constant  Value=acc_mech_trq
  Mux : Mux  Inputs=3
  Product : Product  SaturateOnIntegerOverflow=on
  accessory mechanical torque and power calcs (Nm) : $bdroot/SubLibraries/accessory mechanical torque and power calcs (Nm)
      settings: RTWFcnNameOpts=Auto  RTWFileNameOpts=Auto
  variable mechanical load --simulink implementation-- : $bdroot/SubLibraries/variable mechanical load --simulink implementation--
      settings: RTWFcnNameOpts=Auto  RTWFileNameOpts=Auto
  T_acc : Outport  InitialOutput=0
  P_mech_acc : Outport  Port=2  InitialOutput=0
  wires:
  w_APU/1 -> variable mechanical load --simulink implementation--/1, accessory mechanical torque and power calcs (Nm)/1
  variable mechanical load --simulink implementation--/1 -> Mux/1
  Mux/1 -> accessory mechanical torque and power calcs (Nm)/2
  accessory mechanical torque and power calcs (Nm)/1 -> T_acc/1
  accessory mechanical torque and power calcs (Nm)/2 -> P_mech_acc/1
  Constant2/1 -> Mux/2
  Constant1/1 -> Product/1
  Product/1 -> Mux/3
  [elec_acc_on_bool] -> Product/2

== system lib_accessory2/ACC MECH models/Saber Dual Voltage Cosim ==
  note: (Nm)
  w_APU : Inport
  saber dv acc : Subsystem
  T_acc : Outport  InitialOutput=0
  P_mech_acc : Outport  Port=2  InitialOutput=0
  wires:
  saber dv acc/1(T_acc) -> T_acc/1
  saber dv acc/2(P_acc) -> P_mech_acc/1
  w_APU/1 -> saber dv acc/1(w_APU)

== system lib_accessory2/ACC MECH models/Saber Single Voltage Cosim ==
  note: (Nm)
  w_APU : Inport
  saber sv acc : Subsystem
  T_acc : Outport  InitialOutput=0
  P_mech_acc : Outport  Port=2  InitialOutput=0
  wires:
  w_APU/1 -> saber sv acc/1(w_APU)
  saber sv acc/2(P_acc) -> P_mech_acc/1
  saber sv acc/1(T_acc) -> T_acc/1

== system lib_accessory2/ACC MECH models/SindaTransAC ==
  note: (Nm)
  w_APU : Inport
  accessories (Nm) : Subsystem  mask{sindafile=acc_sindafile}
      mask prompts: sindafile "Path to Sinda\Fluint *.im file"
      mask init:
      | disp(['Sinda Path is ', sindafile])
  T_acc : Outport  InitialOutput=0
  P_mech_acc : Outport  Port=2  InitialOutput=0
  wires:
  accessories (Nm)/1(T_acc) -> T_acc/1
  accessories (Nm)/2(P_acc) -> P_mech_acc/1
  w_APU/1 -> accessories (Nm)/1(w_APU)

== system lib_accessory2/ACC MECH models/mechanical accessories (Nm) ==
  w_APU : Inport
  Mechanical Accessories: Const Mech Var Elect : $bdroot/ACC MECH models/Mechanical Accessories: Const Mech Var Elect
  T_acc : Outport
  P_mech_acc : Outport  Port=2
  wires:
  w_APU/1 -> Mechanical Accessories: Const Mech Var Elect/1
  Mechanical Accessories: Const Mech Var Elect/1 -> T_acc/1
  Mechanical Accessories: Const Mech Var Elect/2 -> P_mech_acc/1

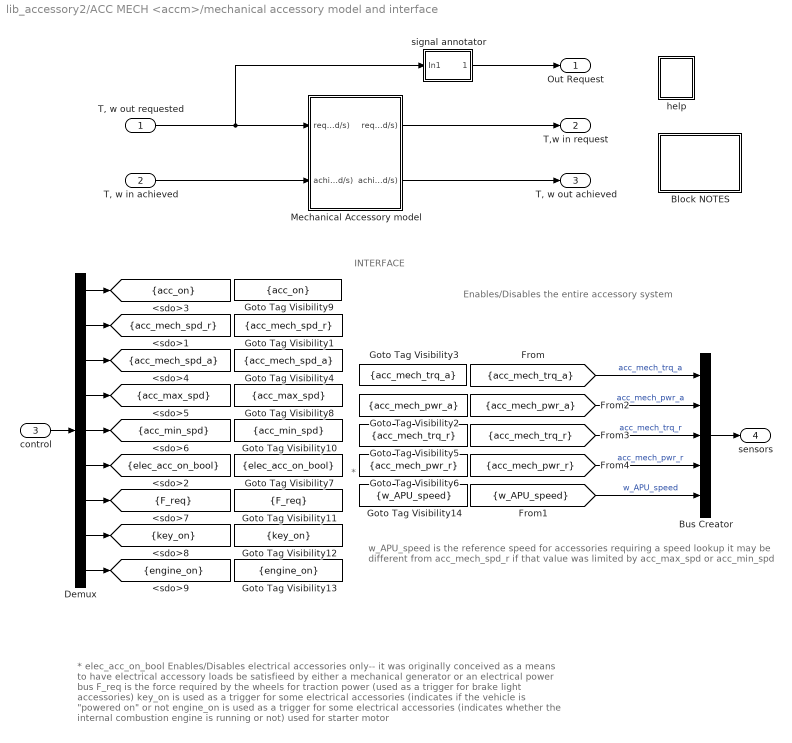
== system lib_accessory2/ACC MECH <accm>/mechanical accessory model and interface ==
  note: INTERFACE
  note: Enables/Disables the entire accessory system
  note: *
  note: * elec_acc_on_bool Enables/Disables electrical accessories only-- it was originally conceived as a means to have electrical accessory loads be
      | satisfieed by either a mechanical generator or an electrical power bus
      |
      | F_req is the force required by the wheels for traction power (used as a trigger for brake light accessories)
      |
      | key_on is used as a trigger for some electrical accessories (indicates if the vehicle is "powered on" or not
      |
      | engine_on is used as a trigger for some electrical accessories (indicates whether the internal combustion engine is running or not) used
      | for starter motor
  note: w_APU_speed is the reference speed for accessories requiring a speed lookup
      | it may be different from acc_mech_spd_r if that value was limited by acc_max_spd
      | or acc_min_spd
  "T, w out requested" : Inport
  "T, w in achieved" : Inport  Port=2
  control : Inport  Port=3
  Block NOTES : Subsystem
      mask Display: disp('Block\nNOTES')
  Bus Creator : BusCreator  Inputs=5
  Demux : Demux  Outputs=9
  Goto Tag Visibility1 : GotoTagVisibility  GotoTag=acc_mech_spd_r
  Goto Tag Visibility10 : GotoTagVisibility  GotoTag=acc_min_spd
  Goto Tag Visibility11 : GotoTagVisibility  GotoTag=F_req
  Goto Tag Visibility12 : GotoTagVisibility  GotoTag=key_on
  Goto Tag Visibility13 : GotoTagVisibility  GotoTag=engine_on
  Goto Tag Visibility14 : GotoTagVisibility  GotoTag=w_APU_speed
  Goto Tag Visibility2 : GotoTagVisibility  GotoTag=acc_mech_pwr_a
  Goto Tag Visibility3 : GotoTagVisibility  GotoTag=acc_mech_trq_a
  Goto Tag Visibility4 : GotoTagVisibility  GotoTag=acc_mech_spd_a
  Goto Tag Visibility5 : GotoTagVisibility  GotoTag=acc_mech_trq_r
  Goto Tag Visibility6 : GotoTagVisibility  GotoTag=acc_mech_pwr_r
  Goto Tag Visibility7 : GotoTagVisibility  GotoTag=elec_acc_on_bool
  Goto Tag Visibility8 : GotoTagVisibility  GotoTag=acc_max_spd
  Goto Tag Visibility9 : GotoTagVisibility  GotoTag=acc_on
  Mechanical Accessory model : Subsystem
      mask Display: image(imread('bdi_acc_pic.bmp'))
  help : Subsystem
      settings: OpenFcn=web(['file:\\\' which('motor_controller.htm')]);
      mask Display: image(imread('doc_man.jpg'))
  signal annotator : Subsystem
  Out Request : Outport
  T,w in request : Outport  Port=2
  "T, w out achieved" : Outport  Port=3
  sensors : Outport  Port=4
  tag scope: F_req=scoped, acc_max_spd=scoped, acc_mech_spd_a=scoped, acc_mech_spd_r=scoped, acc_min_spd=scoped, acc_on=scoped, elec_acc_on_bool=scoped, engine_on=scoped, key_on=scoped
  wires:
  "T, w out requested"/1 -> Mechanical Accessory model/1("requested shaft T and w, out to the driveline  (Nm ; rad/s; rad/s)"), signal annotator/1(In1)
  Mechanical Accessory model/1("requested shaft and belt T and w, in from the prime mover (Nm ; rad/s)") -> T,w in request/1
  "T, w in achieved"/1 -> Mechanical Accessory model/2("achieved shaft and belt T and w, in from the prime mover (Nm ; rad/s)")
  Mechanical Accessory model/2("achieved shaft T and w, out to the driveline (Nm ; rad/s)") -> "T, w out achieved"/1
  Demux/1 -> [acc_on]
  Demux/2 -> [acc_mech_spd_r]
  [acc_mech_trq_a] -> Bus Creator/1  "acc_mech_trq_a"
  [acc_mech_pwr_a] -> Bus Creator/2  "acc_mech_pwr_a"
  [acc_mech_trq_r] -> Bus Creator/3  "acc_mech_trq_r"
  [acc_mech_pwr_r] -> Bus Creator/4  "acc_mech_pwr_r"
  Demux/3 -> [acc_mech_spd_a]
  Demux/4 -> [acc_max_spd]
  Demux/5 -> [acc_min_spd]
  Bus Creator/1 -> sensors/1
  control/1 -> Demux/1
  signal annotator/1(Out1) -> Out Request/1
  Demux/6 -> [elec_acc_on_bool]
  [w_APU_speed] -> Bus Creator/5  "w_APU_speed"
  Demux/7 -> [F_req]
  Demux/8 -> [key_on]
  Demux/9 -> [engine_on]

== system lib_accessory2/Elec Aux Loads 14V Pwr/BrakeLights ==
  Average Watts : Constant  Value=vinf.AuxLoads.BrakeLights.AverageWatts
  Constant : Constant  Value=0
  Constant1 : Constant
  On : Constant  Value=vinf.AuxLoads.BrakeLights.On
  Product : Product  Inputs=4  SaturateOnIntegerOverflow=on
  Switch : Switch  SaturateOnIntegerOverflow=on  InputSameDT=on
  Out1 : Outport
  wires:
  Product/1 -> Out1/1
  Constant/1 -> Switch/1
  [F_req] -> Switch/2
  Constant1/1 -> Switch/3
  Average Watts/1 -> Product/4
  [key_on] -> Product/3
  On/1 -> Product/1
  Switch/1 -> Product/2

== system lib_accessory2/Elec Aux Loads 14V Pwr/Engine ==
  Average Watts : Constant  Value=vinf.AuxLoads.Engine.AverageWatts
  Memory : Memory
  On : Constant  Value=vinf.AuxLoads.Engine.On
  Product : Product  Inputs=4  SaturateOnIntegerOverflow=on
  Out1 : Outport
  wires:
  Memory/1 -> Product/2
  [engine_on] -> Memory/1
  [key_on] -> Product/3
  On/1 -> Product/1
  Product/1 -> Out1/1
  Average Watts/1 -> Product/4

== system lib_accessory2/Elec Aux Loads 14V Pwr/ExternalLights ==
  Average Watts : Constant  Value=vinf.AuxLoads.ExternalLights.AverageWatts
  On : Constant  Value=vinf.AuxLoads.ExternalLights.On
  Product : Product  Inputs=3  SaturateOnIntegerOverflow=on
  Subsystem : lib_cosimulation/Subsystem  ModelName='ExternalLights'
  Out1 : Outport
  wires:
  Average Watts/1 -> Product/3
  On/1 -> Product/1
  Subsystem/1 -> Product/2
  Product/1 -> Out1/1

== system lib_accessory2/Elec Aux Loads 14V Pwr/FrontHVAC ==
  Average Watts : Constant  Value=vinf.AuxLoads.FrontHVAC.AverageWatts
  On : Constant  Value=vinf.AuxLoads.FrontHVAC.On
  Product : Product  Inputs=3  SaturateOnIntegerOverflow=on
  Subsystem : lib_cosimulation/Subsystem  ModelName='FrontHVAC'
  Out1 : Outport
  wires:
  Average Watts/1 -> Product/3
  On/1 -> Product/1
  Subsystem/1 -> Product/2
  Product/1 -> Out1/1

== system lib_accessory2/Elec Aux Loads 14V Pwr/FrontWipers ==
  Average Watts : Constant  Value=vinf.AuxLoads.FrontWipers.AverageWatts
  On : Constant  Value=vinf.AuxLoads.FrontWipers.On
  Product : Product  Inputs=3  SaturateOnIntegerOverflow=on
  Subsystem : lib_cosimulation/Subsystem  ModelName='FrontWipers'
  Out1 : Outport
  wires:
  Average Watts/1 -> Product/3
  On/1 -> Product/1
  Subsystem/1 -> Product/2
  Product/1 -> Out1/1

== system lib_accessory2/Elec Aux Loads 14V Pwr/HeatedSeats ==
  Average Watts : Constant  Value=vinf.AuxLoads.HeatedSeats.AverageWatts
  Num : Constant  Value=vinf.AuxLoads.HeatedSeats.Num
  On : Constant  Value=vinf.AuxLoads.HeatedSeats.On
  Product : Product  Inputs=4  SaturateOnIntegerOverflow=on
  Subsystem : lib_cosimulation/Subsystem  ModelName='HeatedSeats'
  Out1 : Outport
  wires:
  Subsystem/1 -> Product/3
  Product/1 -> Out1/1
  Average Watts/1 -> Product/4
  On/1 -> Product/1
  Num/1 -> Product/2

== system lib_accessory2/Elec Aux Loads 14V Pwr/Misc ==
  Average Watts : Constant  Value=vinf.AuxLoads.Misc.AverageWatts
  On : Constant  Value=vinf.AuxLoads.Misc.On
  Product : Product  Inputs=3  SaturateOnIntegerOverflow=on
  Out1 : Outport
  wires:
  Average Watts/1 -> Product/3
  [key_on] -> Product/2
  On/1 -> Product/1
  Product/1 -> Out1/1

== system lib_accessory2/Elec Aux Loads 14V Pwr/RadiatorCoolingFan ==
  Average Watts : Constant  Value=vinf.AuxLoads.RadiatorCoolingFan.AverageWatts
  On : Constant  Value=vinf.AuxLoads.RadiatorCoolingFan.On
  Product : Product  Inputs=3  SaturateOnIntegerOverflow=on
  Subsystem : lib_cosimulation/Subsystem  ModelName='RadiatorCoolingFan'
  Out1 : Outport
  wires:
  Average Watts/1 -> Product/3
  On/1 -> Product/1
  Subsystem/1 -> Product/2
  Product/1 -> Out1/1

== system lib_accessory2/Elec Aux Loads 14V Pwr/Radio ==
  Average Watts : Constant  Value=vinf.AuxLoads.Radio.AverageWatts
  Num : Constant  Value=vinf.AuxLoads.Radio.Num
  On : Constant  Value=vinf.AuxLoads.Radio.On
  Product : Product  Inputs=4  SaturateOnIntegerOverflow=on
  Subsystem : lib_cosimulation/Subsystem  ModelName='Radio'
  Out1 : Outport
  wires:
  Subsystem/1 -> Product/3
  Average Watts/1 -> Product/4
  On/1 -> Product/1
  Num/1 -> Product/2
  Product/1 -> Out1/1

== system lib_accessory2/Elec Aux Loads 14V Pwr/RearDefrost ==
  Average Watts : Constant  Value=vinf.AuxLoads.RearDefrost.AverageWatts
  On : Constant  Value=vinf.AuxLoads.RearDefrost.On
  Product : Product  Inputs=3  SaturateOnIntegerOverflow=on
  Subsystem : lib_cosimulation/Subsystem  ModelName='RearDefrost'
  Out1 : Outport
  wires:
  Subsystem/1 -> Product/2
  Average Watts/1 -> Product/3
  On/1 -> Product/1
  Product/1 -> Out1/1

== system lib_accessory2/Elec Aux Loads 14V Pwr/RearHVAC ==
  Average Watts : Constant  Value=vinf.AuxLoads.RearHVAC.AverageWatts
  On : Constant  Value=vinf.AuxLoads.RearHVAC.On
  Product : Product  Inputs=3  SaturateOnIntegerOverflow=on
  Subsystem : lib_cosimulation/Subsystem  ModelName='RearHVAC'
  Out1 : Outport
  wires:
  Average Watts/1 -> Product/3
  On/1 -> Product/1
  Subsystem/1 -> Product/2
  Product/1 -> Out1/1

== system lib_accessory2/Elec Aux Loads 14V Pwr/RearWipers ==
  Average Watts : Constant  Value=vinf.AuxLoads.RearWipers.AverageWatts
  On : Constant  Value=vinf.AuxLoads.RearWipers.On
  Product : Product  Inputs=3  SaturateOnIntegerOverflow=on
  Subsystem : lib_cosimulation/Subsystem  ModelName='RearWipers'
  Out1 : Outport
  wires:
  Average Watts/1 -> Product/3
  On/1 -> Product/1
  Subsystem/1 -> Product/2
  Product/1 -> Out1/1
